simulink model "MAS_Full_State_AS"  (R2021b)
settings: Solver=VariableStepAuto  StartTime=0.0  StopTime=50  RelTol=1e-3
libraries: cstblocks x6
settings Model: Creator=lenovo  LastModifiedBy=lenovo

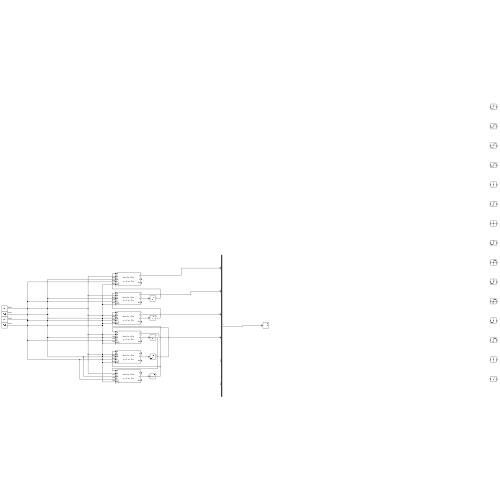
[thumbnail: Simulink's stored preview of the top-level diagram]
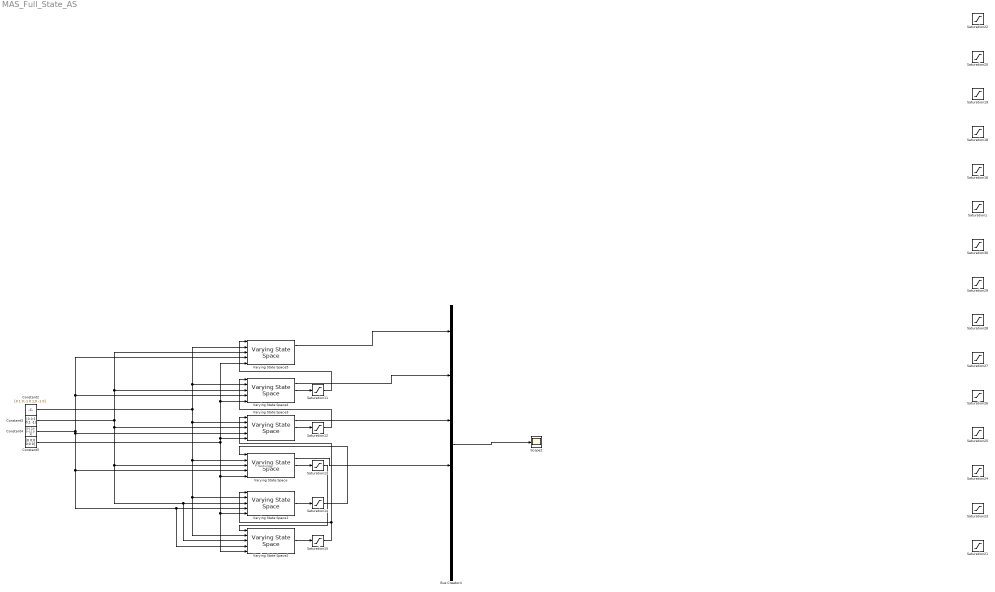
== system MAS_Full_State_AS ==
  note: P resburger
  Bus Creator4 : BusCreator  Inputs=6
  Constant2 : Constant  Value=[0 1 0;-1 0 1;0 -1 0]
  Constant3 : Constant  Value=[0 0;1 0;1 -1]
  Constant4 : Constant  Value=[0 1 2;0 0 -1;1 0 1]  VectorParams1D=off
  Constant5 : Constant  Value=[0 0;0 0;0 0]  VectorParams1D=off
  Saturation{1,16,18..30} (15 alike) : Saturate  UpperLimit=1  LowerLimit=-1
  Saturation{11..15} (5 alike) : Saturate  UpperLimit=0.05  LowerLimit=-0.05
  Scope2 : Scope
  Varying State Space{,1,3..5} (5 alike) : cstblocks/Linear Parameter Varying/Varying State Space  x0=0  xNames=''  OutputX=on  OutputDX=on
  Varying State Space2 : cstblocks/Linear Parameter Varying/Varying State Space  x0=[1;0;0;0]  xNames=''  OutputX=on  OutputDX=on
  wires:
  Bus Creator4/1 -> Scope2/1
  Varying State Space2/2 -> Saturation15/1
  Varying State Space1/2 -> Saturation14/1
  Varying State Space/2 -> Saturation13/1
  Varying State Space3/2 -> Saturation12/1
  Varying State Space4/2 -> Saturation11/1
  Constant2/1 -> Varying State Space2/2, Varying State Space1/2, Varying State Space/2, Varying State Space3/2, Varying State Space4/2, Varying State Space5/2
  Constant3/1 -> Varying State Space3/3, Varying State Space2/3, Varying State Space1/3, Varying State Space/3, Varying State Space4/3, Varying State Space5/3
  Constant4/1 -> Varying State Space/4, Varying State Space2/4, Varying State Space1/4, Varying State Space3/4, Varying State Space4/4, Varying State Space5/4
  Constant5/1 -> Varying State Space/5, Varying State Space2/5, Varying State Space1/5, Varying State Space5/5, Varying State Space4/5, Varying State Space3/5
  Saturation15/1 -> Varying State Space3/1, Varying State Space1/1
  Saturation14/1 -> Varying State Space/1
  Saturation13/1 -> Varying State Space2/1
  Saturation12/1 -> Varying State Space4/1
  Saturation11/1 -> Varying State Space5/1
  Varying State Space5/1 -> Bus Creator4/1
  Varying State Space4/1 -> Bus Creator4/2
  Varying State Space3/1 -> Bus Creator4/3
  Varying State Space/1 -> Bus Creator4/4
